simulink model "Led_photo_transZ_3"  (Simulink 7.4)
settings: Solver=ode45  StartTime=0.0  StopTime=1e-5  RelTol=1e-3
libraries: powerlib x18, commrandsrc2 x1, simulink x1
settings Model: Creator=dbenson  LastModifiedBy=Dick
settings SolverCC: InitialStep=1e-9
settings DataIOCC: SignalLoggingName=sigsOut
settings OptimizationCC: InlineInvariantSignals=on  InitFltsAndDblsToZero=on
settings DebuggingCC: SaveWithParameterizedLinksMsg=none  SignalResolutionControl=TryResolveAllWithWarning  SolverPrmCheckMsg=none  MultiTaskDSMMsg=warning  MultiTaskCondExecSysMsg=none  StrictBusMsg=None
settings HardwareCC: TargetUnknown=on
settings RTWCC: IncludeERTFirstTime=on
settings GRTTargetCC: TargetFcnLib=ansi_tfl_tmw.mat

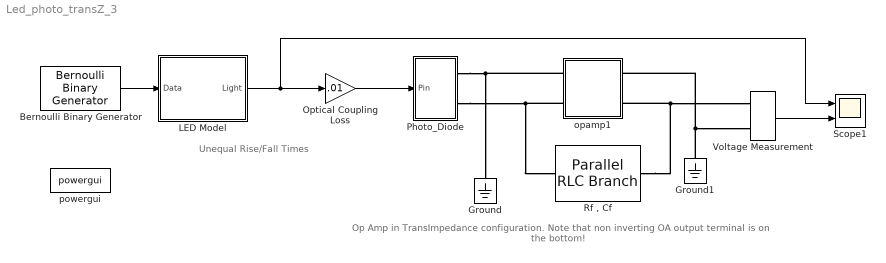
== system Led_photo_transZ_3 ==
  note: Op Amp in TransImpedance configuration.
      | Note that non inverting OA output terminal is on the bottom!
  note: Unequal Rise/Fall Times
  Bernoulli Binary Generator : commrandsrc2/Bernoulli Binary Generator  DialogController=commDDGCreate  DialogControllerArgs=DataTag0  SystemSampleTime=-1  P=0.5  seed=61  Ts=1/100e6  frameBased=off  sampPerFrame=1  orient=off  outDataType=double
  Ground : powerlib/Elements/Ground  DialogController=POWERSYS.PowerSysDialog  PhysicalDomain=powersysdomain  SubClassName=unknown  LeftPortType=p1  RightPortType=p1  LConnTagsString=a
  Ground1 : powerlib/Elements/Ground  DialogController=POWERSYS.PowerSysDialog  PhysicalDomain=powersysdomain  SubClassName=unknown  LeftPortType=p1  RightPortType=p1  LConnTagsString=a
  LED Model : Subsystem
  Optical Coupling Loss : Gain  Gain=.01  ParameterDataType=sfix(16)  ParameterScaling=2^0  OutDataType=sfix(16)  OutScaling=2^0
  Photo_Diode : Subsystem  mask{Sens=5, Cout=20e-12, Rout=1e3}
      mask prompts: Sens "Sensitivity in A/W"; Cout "Output Capacitance"; Rout "Output Resistance"
  "Rf , Cf" : powerlib/Elements/Parallel RLC Branch  DialogController=POWERSYS.PowerSysDialog  PhysicalDomain=powersysdomain  SubClassName=unknown  LeftPortType=p1  RightPortType=p1  LConnTagsString=a  RConnTagsString=__new0  BranchType=RC  Resistance=10000  Inductance=1.0  SetiL0=off  InitialCurrent=0  Capacitance=.5e-12  Setx0=off  InitialVoltage=0  Measurements=None
  Scope1 : Scope  NumInputPorts=2
      settings: TimeRange=1.2e-005  YMin=-0.0005~-1  YMax=0.003~2
  Voltage Measurement : powerlib/Measurements/Voltage Measurement  Tag=PoWeRsYsTeMmEaSuReMeNt  DialogController=POWERSYS.PowerSysDialog  SystemSampleTime=-1  PhasorSimulation=off  OutputType=Magnitude  PSBequivalent=0
  opamp1 : Subsystem  mask{f2=1e7, f1=1e8, Av=400, Ro=1000, v_min=-3, v_max=3, slew_rate=40e9}
      mask prompts: f2 "break freq 2 in Hz"; f1 "break freq 1 in Hz"; Av "Av (voltage gain)"; Ro "Output Resistance"; v_min "Min Output"; v_max "Max Output"; slew_rate "slew rate (v/s)"
      mask Display: plot([0 1 0 0] , [1 0 -1 1 ]); text(0.15,0.4,'+'); text(0.15,-0.4,'-');
  powergui : powerlib/powergui  SystemSampleTime=-1  SimulationMode=Continuous  SampleTime=0  frequency=60  SPID=off  DisableSnubberDevices=off  DisableRonSwitches=off  DisableVfSwitches=off  SwTol=0  Interpol=off  frequencyindice=0  echomessages=off  HookPort=off  DisplayEquations=off  FunctionMessages=off  EnableUseOfTLC=off  x0status=blocks  RestoreLinks=warning  Frange=[0:2:500]  Ylog=off  Xlog=on  ShowGrid=off  save=off  variable=ZData  ZoomFFT=on  StartTime=0.0  cycles=1  DisplayStyle=1  fundamental=60  FreqAxis=off  MaxFrequency=1000  frequencyindicesteady=1  RmsSteady=1  display=off  Ts=0  methode=off
  wires:
  Optical Coupling Loss/1 -> Photo_Diode/1(Pin)
  Voltage Measurement/1 -> Scope1/2
  LED Model/1(Light) -> Optical Coupling Loss/1, Scope1/1
  Bernoulli Binary Generator/1 -> LED Model/1(Data)
  connections:
  opamp1/RConn2 -- "Rf , Cf"/RConn1 -- Voltage Measurement/LConn1
  opamp1/RConn1 -- Ground1/LConn1 -- Voltage Measurement/LConn2
  opamp1/LConn2 -- "Rf , Cf"/LConn1 -- Photo_Diode/RConn2
  opamp1/LConn1 -- Ground/LConn1 -- Photo_Diode/RConn1

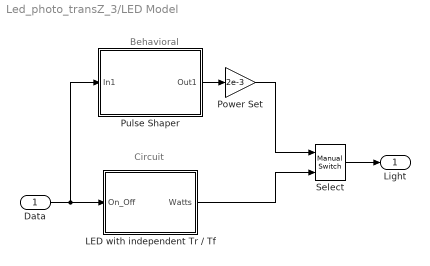
== system Led_photo_transZ_3/LED Model ==
  note: Behavioral
  note: Circuit
  Data : Inport
  LED with independent Tr / Tf : Subsystem  mask{Watts=2e-3, Tr=2e-9, Tf=0.5e-9}
      mask prompts: Tr "Rise Time"; Tf "Fall time (Tf <=Tr)"
  Power Set : Gain  Gain=2e-3  ParameterDataType=sfix(16)  ParameterScaling=2^0  OutDataType=sfix(16)  OutScaling=2^0
  Pulse Shaper : Subsystem  mask{Tr=2e-9, Tf=0.5e-9, Vofs=.5}
      mask prompts: Tr "Rise Time"; Tf "Fall Time"; Vofs "Offset"
      mask Display: disp('Pulse Shaper')
  Select : simulink/Signal Routing/Manual Switch  SystemSampleTime=-1  sw=1  action=0  varsize=off
  Light : Outport
  wires:
  Pulse Shaper/1(Out1) -> Power Set/1
  LED with independent Tr / Tf/1(Watts) -> Select/2
  Power Set/1 -> Select/1
  Select/1 -> Light/1
  Data/1 -> LED with independent Tr / Tf/1(On_Off), Pulse Shaper/1(In1)

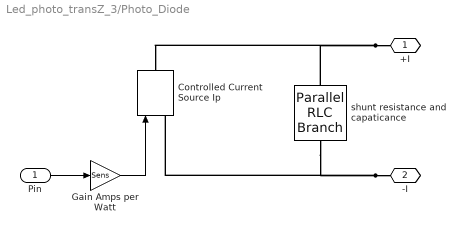
== system Led_photo_transZ_3/Photo_Diode ==
  Pin : Inport
  Controlled Current Source Ip : powerlib/Electrical Sources/Controlled Current Source  DialogController=POWERSYS.PowerSysDialog  SystemSampleTime=-1  Initialize=off  Source_Type=DC  Amplitude=0  Phase=0  Frequency=0  Measurements=None
  Gain Amps per Watt : Gain  Gain=Sens  ParameterDataType=sfix(16)  ParameterScaling=2^0  OutDataType=sfix(16)  OutScaling=2^0
  shunt resistance and  capaticance : powerlib/Elements/Parallel RLC Branch  DialogController=POWERSYS.PowerSysDialog  PhysicalDomain=powersysdomain  SubClassName=unknown  LeftPortType=p1  RightPortType=p1  LConnTagsString=a  RConnTagsString=__new0  BranchType=RC  Resistance=Rout  Inductance=1e-3  SetiL0=off  InitialCurrent=0  Capacitance=Cout  Setx0=off  InitialVoltage=0  Measurements=None
  +I : PMIOPort  Port=1  Side=Right
  -I : PMIOPort  Port=2  Side=Right
  wires:
  Gain Amps per Watt/1 -> Controlled Current Source Ip/1
  Pin/1 -> Gain Amps per Watt/1
  connections:
  -I/RConn1 -- shunt resistance and  capaticance/RConn1 -- Controlled Current Source Ip/LConn1
  +I/RConn1 -- shunt resistance and  capaticance/LConn1 -- Controlled Current Source Ip/RConn1

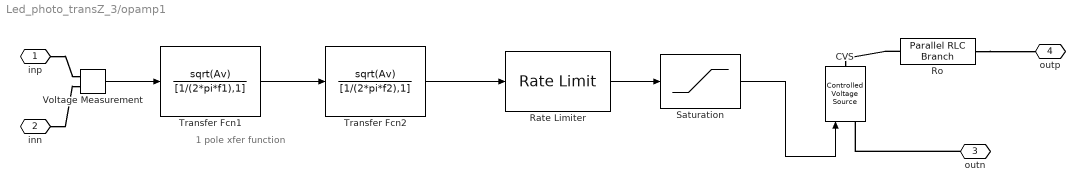
== system Led_photo_transZ_3/opamp1 ==
  note: 1 pole xfer function
  CVS : powerlib/Electrical Sources/Controlled Voltage Source  Description=source block  DialogController=POWERSYS.PowerSysDialog  SystemSampleTime=-1  Initialize=off  Source_Type=AC  Amplitude=0  Phase=0  Frequency=0  Measurements=None
      settings: AttributesFormatString=\n
  Rate Limiter : RateLimiter  RisingSlewLimit=slew_rate  FallingSlewLimit=-slew_rate  LinearizeAsGain=off
  Ro : powerlib/Elements/Parallel RLC Branch  DialogController=POWERSYS.PowerSysDialog  PhysicalDomain=powersysdomain  SubClassName=unknown  LeftPortType=p1  RightPortType=p1  LConnTagsString=a  RConnTagsString=__new0  BranchType=R  Resistance=Ro  Inductance=1.0  SetiL0=off  InitialCurrent=0  Capacitance=200e-12  Setx0=off  InitialVoltage=0  Measurements=None
  Saturation : Saturate  UpperLimit=v_max  LowerLimit=v_min  LinearizeAsGain=off  ZeroCross=off
  Transfer Fcn1 : TransferFcn  Numerator=sqrt(Av)  Denominator=[1/(2*pi*f1),1]
  Transfer Fcn2 : TransferFcn  Numerator=sqrt(Av)  Denominator=[1/(2*pi*f2),1]
  Voltage Measurement : powerlib/Measurements/Voltage Measurement  Tag=PoWeRsYsTeMmEaSuReMeNt  DialogController=POWERSYS.PowerSysDialog  SystemSampleTime=-1  PhasorSimulation=off  OutputType=Magnitude  PSBequivalent=0
  inp : PMIOPort  Port=1  Side=Left
  inn : PMIOPort  Port=2  Side=Left
  outn : PMIOPort  Port=3  Side=Right
  outp : PMIOPort  Port=4  Side=Right
  wires:
  Voltage Measurement/1 -> Transfer Fcn1/1
  Rate Limiter/1 -> Saturation/1
  Transfer Fcn1/1 -> Transfer Fcn2/1
  Saturation/1 -> CVS/1
  Transfer Fcn2/1 -> Rate Limiter/1
  connections:
  outn/RConn1 -- CVS/LConn1
  inn/RConn1 -- Voltage Measurement/LConn2
  inp/RConn1 -- Voltage Measurement/LConn1
  Ro/LConn1 -- CVS/RConn1
  Ro/RConn1 -- outp/RConn1

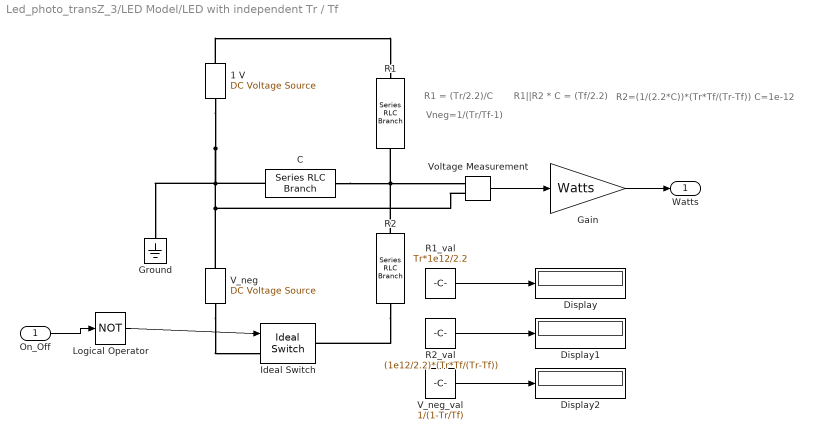
== system Led_photo_transZ_3/LED Model/LED with independent Tr / Tf ==
  note: R1 = (Tr/2.2)/C
  note: R1||R2 * C = (Tf/2.2)
  note: C=1e-12
  note: R2=(1/(2.2*C))*(Tr*Tf/(Tr-Tf))
  note: Vneg=1/(Tr/Tf-1)
  On_Off : Inport
  " 1 V" : powerlib/Electrical Sources/DC Voltage Source  DialogController=POWERSYS.PowerSysDialog  SystemSampleTime=-1  Amplitude=1  Measurements=None
  " V_neg" : powerlib/Electrical Sources/DC Voltage Source  DialogController=POWERSYS.PowerSysDialog  SystemSampleTime=-1  Amplitude=1/(Tr/Tf-1)  Measurements=None
  C : powerlib/Elements/Series RLC Branch  DialogController=POWERSYS.PowerSysDialog  PhysicalDomain=powersysdomain  SubClassName=unknown  LeftPortType=p1  RightPortType=p1  LConnTagsString=__new0  RConnTagsString=__new0  BranchType=C  Resistance=1  Inductance=1e-3  SetiL0=off  InitialCurrent=0  Capacitance=1e-12  Setx0=on  InitialVoltage=0  Measurements=None
  Display : Display
  Display1 : Display
  Display2 : Display
  Gain : Gain  Gain=Watts  ParameterDataType=sfix(16)  ParameterScaling=2^0  OutDataType=sfix(16)  OutScaling=2^0
  Ground : powerlib/Elements/Ground  DialogController=POWERSYS.PowerSysDialog  PhysicalDomain=powersysdomain  SubClassName=unknown  LeftPortType=p1  RightPortType=p1  LConnTagsString=a
  Ideal Switch : powerlib/Power Electronics/Ideal Switch  DialogController=POWERSYS.PowerSysDialog  SystemSampleTime=-1  Ron=.001  Lon=0  IC=0  Rs=inf  Cs=0  Measurements=off
  Logical Operator : Logic  Operator=NOT  AllPortsSameDT=off  OutDataTypeMode=boolean  LogicDataType=fixdt(0, 8)  OutDataTypeStr=boolean
  R1 : powerlib/Elements/Series RLC Branch  DialogController=POWERSYS.PowerSysDialog  PhysicalDomain=powersysdomain  SubClassName=unknown  LeftPortType=p1  RightPortType=p1  LConnTagsString=__new0  RConnTagsString=__new0  BranchType=R  Resistance=Tr*1e12/2.2  Inductance=1e-3  SetiL0=off  InitialCurrent=0  Capacitance=1e-6  Setx0=off  InitialVoltage=0  Measurements=None
  R1_val : Constant  Value=Tr*1e12/2.2  OutDataType=sfix(16)  OutScaling=2^0
  R2 : powerlib/Elements/Series RLC Branch  DialogController=POWERSYS.PowerSysDialog  PhysicalDomain=powersysdomain  SubClassName=unknown  LeftPortType=p1  RightPortType=p1  LConnTagsString=__new0  RConnTagsString=__new0  BranchType=R  Resistance=(1e12*(Tr*Tf/(Tr-Tf)))/2.2  Inductance=1e-3  SetiL0=off  InitialCurrent=0  Capacitance=1e-6  Setx0=off  InitialVoltage=0  Measurements=None
  R2_val : Constant  Value=(1e12/2.2)*(Tr*Tf/(Tr-Tf))  OutDataType=sfix(16)  OutScaling=2^0
  V_neg_val : Constant  Value=1/(1-Tr/Tf)  OutDataType=sfix(16)  OutScaling=2^0
  Voltage Measurement : powerlib/Measurements/Voltage Measurement  DialogController=POWERSYS.PowerSysDialog  SystemSampleTime=-1  PhasorSimulation=off  OutputType=Complex  PSBequivalent=0
  Watts : Outport
  wires:
  On_Off/1 -> Logical Operator/1
  Gain/1 -> Watts/1
  Voltage Measurement/1 -> Gain/1
  R1_val/1 -> Display/1
  R2_val/1 -> Display1/1
  V_neg_val/1 -> Display2/1
  Logical Operator/1 -> Ideal Switch/1
  connections:
  " 1 V"/RConn1 -- R1/LConn1
  Voltage Measurement/LConn2 -- C/RConn1 -- " 1 V"/LConn1 -- Ground/LConn1 -- " V_neg"/RConn1
  R2/LConn1 -- C/LConn1 -- R1/RConn1 -- Voltage Measurement/LConn1
  R2/RConn1 -- Ideal Switch/RConn1
  " V_neg"/LConn1 -- Ideal Switch/LConn1

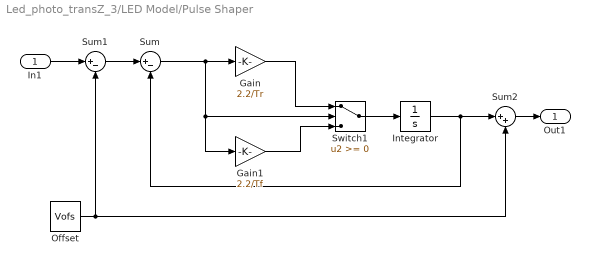
== system Led_photo_transZ_3/LED Model/Pulse Shaper ==
  In1 : Inport
  Gain : Gain  Gain=2.2/Tr  ParameterDataType=sfix(16)  ParameterScaling=2^0  OutDataType=sfix(16)  OutScaling=2^0
  Gain1 : Gain  Gain=2.2/Tf  ParameterDataType=sfix(16)  ParameterScaling=2^0  OutDataType=sfix(16)  OutScaling=2^0
  Integrator : Integrator
  Offset : Constant  Value=Vofs  OutDataType=fixdt(1, 16)  OutScaling=2^0
  Sum : Sum  Inputs=|+-  OutDataType=sfix(16)  OutScaling=2^0
  Sum1 : Sum  Inputs=|+-  OutDataType=sfix(16)  OutScaling=2^0
  Sum2 : Sum  Inputs=|++  OutDataType=sfix(16)  OutScaling=2^0
  Switch1 : Switch
  Out1 : Outport
  wires:
  Integrator/1 -> Sum/2, Sum2/1
  Sum/1 -> Gain/1, Gain1/1, Switch1/2
  Gain/1 -> Switch1/1
  Gain1/1 -> Switch1/3
  Switch1/1 -> Integrator/1
  Sum1/1 -> Sum/1
  Offset/1 -> Sum1/2, Sum2/2
  In1/1 -> Sum1/1
  Sum2/1 -> Out1/1
